simulink library "Battery_EB"  (R2018b)
settings: Solver=ode45  StartTime=0.0  StopTime=10.0  RelTol=1e-3  EnableMultiTasking=on
undefined symbols (not defined in the file): dummy
libraries: carnot x2
settings Model: Creator=lena.frank  LastModifiedBy=drhf
settings DataIOCC: LimitDataPoints=on  SaveFormat=Array  SignalLoggingSaveFormat=ModelDataLogs
settings OptimizationCC: ExpressionDepthLimit=2147483647  LifeSpan=inf
settings DebuggingCC: UnderspecifiedInitializationDetection=Classic  MergeDetectMultiDrivingBlocksExec=none  SolverPrmCheckMsg=warning  FcnCallInpInsideContextMsg=warning  StateNameClashWarn=warning  SFUnexpectedBacktrackingDiag=warning  SFNoUnconditionalDefaultTransitionDiag=warning  SFExecutionAtInitializationDiag=none
settings HardwareCC: ProdBitPerPointer=32  ProdBitPerSizeT=32  ProdBitPerPtrDiffT=32  ProdLargestAtomicFloat=None  ProdIntDivRoundTo=Undefined  ProdEndianess=Unspecified  ProdWordSize=32  ProdHWDeviceType=32-bit Generic
settings ModelReferenceCC: PropagateSignalLabelsOutOfModel=off
settings SFSimCC: SimUseLocalCustomCode=off
settings RTWCC: RTWUseLocalCustomCode=off
settings CodeAppCC: StateflowObjectComments=on
settings GRTTargetCC: TargetLangStandard=C89/C90 (ANSI)  GeneratePreprocessorConditionals=Disable all  CombineOutputUpdateFcns=off  GRTInterface=on
settings ConfigComp: CovMetricSettings=dw  CovHtmlReporting=on  CovSaveCumulativeToWorkspaceVar=on  CovSaveSingleToWorkspaceVar=on  CovExternalEMLEnable=off

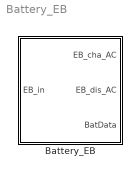
== system Battery_EB ==
  Battery_EB : Subsystem  TreatAsAtomicUnit=on  mask(electric Battery){cap_kWh=5e6/3.6e6, eta_ch=0.9, eta_dis=0.9, cap0=1, SOC_max=1, SOC_min=0, Pmax=1000, Pmin=1000, P_standby=10}
      mask prompts: cap_kWh "Capacity in kWh"; eta_ch "Charging efficiency"; eta_dis "Discharging efficiency"; cap0 "Initial charge condition (0...1)"; SOC_max "Maximal SOC [-]"; SOC_min "Minimal SOC [-]"; Pmax "Maximal input power"; Pmin "Maximal output power"; P_standby "Standby power consumption [W]"
      mask help:
      | Electric energy storage ('rechargable battery') with inverter, based on an energy balance.
      | dE/dt = P_in * efficiency
      | The model uses a single phase connection (ActPower1 in EB_in). Separate parameters are used for charging and discharging efficiency.
      | Negative power at inport EB_in is for discharging, positive vor charging.
      | If the battery is full, the power is led to the output P_over (in BatData).
      | If the battery is emtpty, the missing power is led to the output P_under (in BatData).
      | The state output gives the state of charge in 0...1.
      mask init:
      | capa = cap_kWh*1e3*3600;
      | Pmax = abs(Pmax);
      | Pmin = abs(Pmin);
      settings: MinAlgLoopOccurrences=on
      mask Help: web(fullfile(path_carnot('help'),'Battery.html'),'-helpbrowser')
      mask Display: plot(0,-10,120,100,[70,70,60,40,30,30,40,60,70,60,40,30],[80,10,-0,-0,10,80,70,70,80,90,90,80],[44,47,54,57,54,47,44],[80,76,76,80,84,84,80])

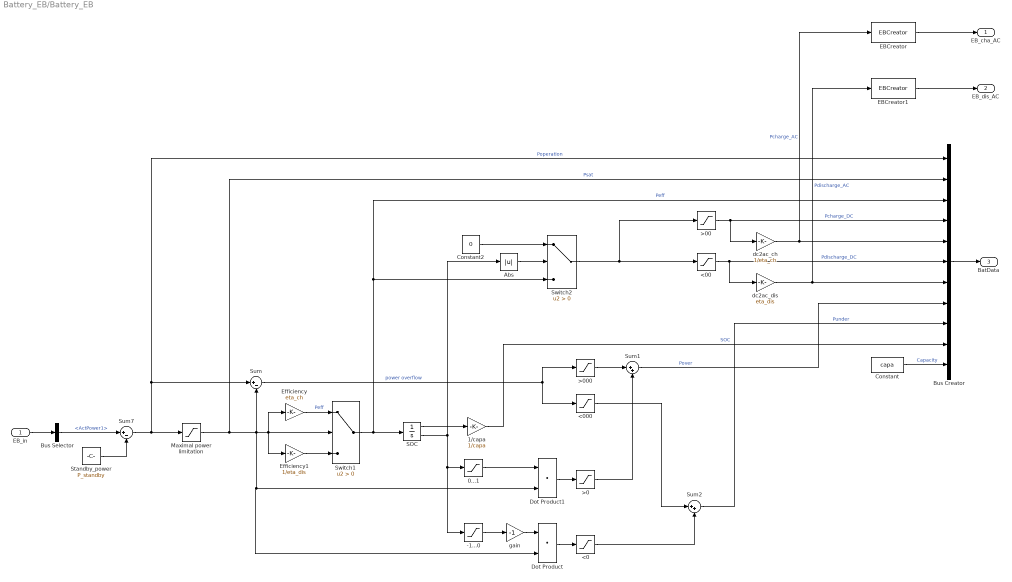
== system Battery_EB/Battery_EB ==
  EB_in : Inport
  -1...0 : Saturate  UpperLimit=0  LowerLimit=-1
  0...1 : Saturate  UpperLimit=1  LowerLimit=0
  1/capa : Gain  Gain=1/capa
  <0 : Saturate  UpperLimit=0  LowerLimit=-inf
  <00 : Saturate  UpperLimit=0  LowerLimit=-inf
  <000 : Saturate  UpperLimit=0  LowerLimit=-inf
  >0 : Saturate  UpperLimit=inf  LowerLimit=0
  >00 : Saturate  UpperLimit=inf  LowerLimit=0
  >000 : Saturate  UpperLimit=inf  LowerLimit=0
  Abs : Abs
  Bus Creator : BusCreator  Inputs=11
  Bus Selector : BusSelector  OutputSignals=ActPower1
  Constant : Constant  Value=capa
  Constant2 : Constant  Value=0
  Dot Product : DotProduct  InputSameDT=on  OutDataTypeStr=Inherit: Inherit via internal rule
  Dot Product1 : DotProduct  InputSameDT=on  OutDataTypeStr=Inherit: Inherit via internal rule
  EBCreator : carnot/Basic/Electric/EBCreator  Inport_ID=off  Inport_f=off  Inport_v1=off  Inport_p1=on  Inport_pf1=off  Inport_v2=off  Inport_p2=off  Inport_pf2=off  Inport_v3=off  Inport_p3=off  Inport_pf3=off  ID=1  f=0  v1=400%dummy  p1=1e5  pf1=1  v2=0  p2=1e5  pf2=1  v3=0  p3=0  pf3=1  Annotation_ID=on  Annotation_f=on  Annotation_v1=on  Annotation_p1=off  Annotation_pf1=off  Annotation_v2=off  Annotation_p2=off  Annotation_pf2=off  Annotation_v3=off  Annotation_p3=off  Annotation_pf3=off
      settings: SourceProductName=Carnot
      settings: AttributesFormatString=|
      | ID 1
      | 0 Hz frequency
      | 400%dummy V Voltage
  EBCreator1 : carnot/Basic/Electric/EBCreator  Inport_ID=off  Inport_f=off  Inport_v1=off  Inport_p1=on  Inport_pf1=off  Inport_v2=off  Inport_p2=off  Inport_pf2=off  Inport_v3=off  Inport_p3=off  Inport_pf3=off  ID=1  f=0  v1=400%dummy  p1=1e5  pf1=1  v2=0  p2=1e5  pf2=1  v3=0  p3=0  pf3=1  Annotation_ID=on  Annotation_f=on  Annotation_v1=on  Annotation_p1=off  Annotation_pf1=off  Annotation_v2=off  Annotation_p2=off  Annotation_pf2=off  Annotation_v3=off  Annotation_p3=off  Annotation_pf3=off
      settings: SourceProductName=Carnot
      settings: AttributesFormatString=|
      | ID 1
      | 0 Hz frequency
      | 400%dummy V Voltage
  Efficiency : Gain  Gain=eta_ch
  Efficiency1 : Gain  Gain=1/eta_dis
  Maximal power limitation : Saturate  UpperLimit=Pmax/eta_ch  LowerLimit=-Pmin*eta_dis
  SOC : Integrator  InitialCondition=cap0*capa  LimitOutput=on  UpperSaturationLimit=SOC_max*capa  LowerSaturationLimit=SOC_min*capa  ShowSaturationPort=on
  Standby_power : Constant  Value=P_standby
  Sum : Sum  Inputs=|+-
  Sum1 : Sum  Inputs=|++
  Sum2 : Sum  Inputs=|++
  Sum7 : Sum  Inputs=|+-
  Switch1 : Switch  Criteria=u2 > Threshold
  Switch2 : Switch  Criteria=u2 > Threshold
  dc2ac_ch : Gain  Gain=1/eta_ch
  dc2ac_dis : Gain  Gain=eta_dis
  gain : Gain  Gain=-1
  EB_cha_AC : Outport
  EB_dis_AC : Outport  Port=2
  BatData : Outport  Port=3
  wires:
  Constant/1 -> Bus Creator/11  "Capacity"
  Bus Selector/1 -> Sum7/1  "<ActPower1>"
  EB_in/1 -> Bus Selector/1
  >00/1 -> dc2ac_ch/1, Bus Creator/4  "Pcharge_DC"
  Sum2/1 -> Bus Creator/9  "Punder"
  Bus Creator/1 -> BatData/1
  <00/1 -> dc2ac_dis/1, Bus Creator/6  "Pdischarge_DC"
  <000/1 -> Sum2/1
  <0/1 -> Sum2/2
  >000/1 -> Sum1/1
  >0/1 -> Sum1/2
  Sum/1 -> <000/1, >000/1  "power overflow"
  Maximal power limitation/1 -> Sum/2, Dot Product/2, Dot Product1/2, Switch1/2, Efficiency1/1, Efficiency/1, Bus Creator/2  "Psat"
  SOC/1 -> 1/capa/1
  1/capa/1 -> Bus Creator/10  "SOC"
  SOC/2 -> Abs/1, 0...1/1, -1...0/1
  gain/1 -> Dot Product/1
  Dot Product/1 -> <0/1
  -1...0/1 -> gain/1
  0...1/1 -> Dot Product1/1
  Dot Product1/1 -> >0/1
  Switch1/1 -> SOC/1, Switch2/3, Bus Creator/3  "Peff"
  Standby_power/1 -> Sum7/2
  Efficiency/1 -> Switch1/1  "Peff"
  Efficiency1/1 -> Switch1/3
  Switch2/1 -> <00/1, >00/1
  Abs/1 -> Switch2/2
  Constant2/1 -> Switch2/1
  Sum7/1 -> Maximal power limitation/1, Sum/1, Bus Creator/1  "Poperation"
  Sum1/1 -> Bus Creator/8  "Pover"
  dc2ac_ch/1 -> EBCreator/1, Bus Creator/5  "Pcharge_AC"
  dc2ac_dis/1 -> EBCreator1/1, Bus Creator/7  "Pdischarge_AC"
  EBCreator1/1 -> EB_dis_AC/1
  EBCreator/1 -> EB_cha_AC/1
